simulink model "modos_deslizantes"  (R2025b)
settings: Solver=VariableStepAuto  StartTime=0.0  StopTime=50  RelTol=1e-3
libraries: simulink x1
settings Model: Creator=LENOVO  LastModifiedBy=LENOVO

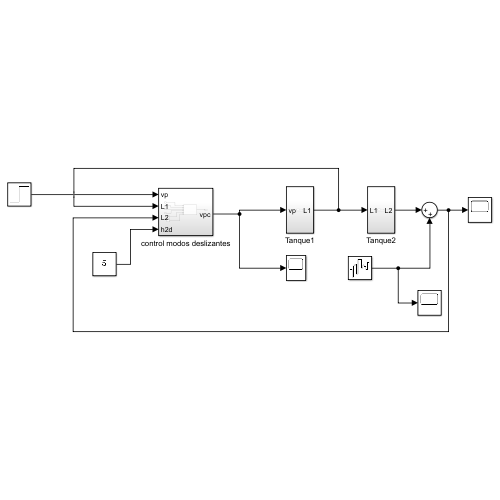
[thumbnail: Simulink's stored preview of the top-level diagram]
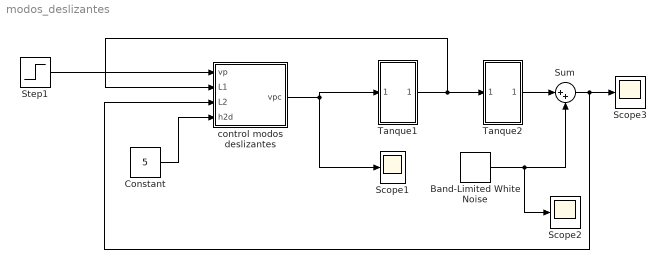
== system modos_deslizantes ==
  Band-Limited White Noise : simulink/Sources/Band-Limited White Noise  Cov=[0.1]  Ts=5  seed=[23341]
  Constant : Constant  Value=5
  Scope1 : Scope
      settings: ActiveDisplayYMinimum=-29.991396434772103  ActiveDisplayYMaximum=28.288118686222941
  Scope2 : Scope
      settings: ActiveDisplayYMinimum=-3.4612563380497452  ActiveDisplayYMaximum=7.7257857094803253  DataLoggingVariableName=ScopeData2
  Scope3 : Scope
      settings: ActiveDisplayYMinimum=-3.4612563380497452  ActiveDisplayYMaximum=7.7257857094803253
  Step1 : Step  After=8  SampleTime=0
  Sum : Sum  Inputs=|++
  Tanque1 : Subsystem
  Tanque2 : Subsystem
  control modos deslizantes : Subsystem
  wires:
  Band-Limited White Noise/1 -> Sum/2, Scope2/1
  control modos deslizantes/1(vpc) -> Tanque1/1(vp), Scope1/1
  Tanque2/1(L2) -> Sum/1
  Sum/1 -> Scope3/1, control modos deslizantes/3(L2)
  Step1/1 -> control modos deslizantes/1(vp)
  Tanque1/1(L1) -> control modos deslizantes/2(L1), Tanque2/1(L1)
  Constant/1 -> control modos deslizantes/4(h2d)

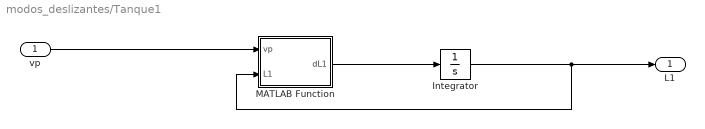
== system modos_deslizantes/Tanque1 ==
  vp : Inport
  Integrator : Integrator
  MATLAB Function : MATLAB Function  TreatAsAtomicUnit=on
  L1 : Outport
  wires:
  Integrator/1 -> L1/1, MATLAB Function/2(L1)
  MATLAB Function/1(dL1) -> Integrator/1
  vp/1 -> MATLAB Function/1(vp)

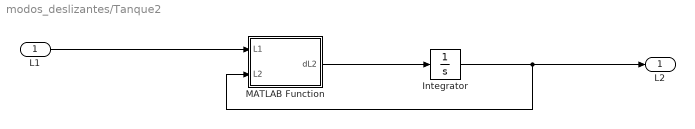
== system modos_deslizantes/Tanque2 ==
  L1 : Inport
  Integrator : Integrator
  MATLAB Function : MATLAB Function  TreatAsAtomicUnit=on
  L2 : Outport
  wires:
  Integrator/1 -> MATLAB Function/2(L2), L2/1
  MATLAB Function/1(dL2) -> Integrator/1
  L1/1 -> MATLAB Function/1(L1)

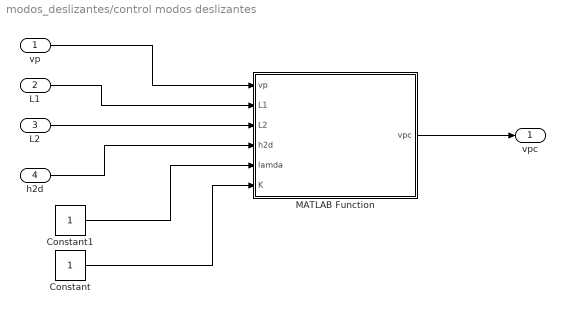
== system modos_deslizantes/control modos deslizantes ==
  vp : Inport
  L1 : Inport  Port=2
  L2 : Inport  Port=3
  h2d : Inport  Port=4
  Constant : Constant
  Constant1 : Constant
  MATLAB Function : MATLAB Function  TreatAsAtomicUnit=on
  vpc : Outport
  wires:
  L1/1 -> MATLAB Function/2(L1)
  MATLAB Function/1(vpc) -> vpc/1
  L2/1 -> MATLAB Function/3(L2)
  vp/1 -> MATLAB Function/1(vp)
  Constant1/1 -> MATLAB Function/5(lamda)
  Constant/1 -> MATLAB Function/6(K)
  h2d/1 -> MATLAB Function/4(h2d)

== matlab function modos_deslizantes/Tanque2/MATLAB Function ==
  data: L1 input; L2 input; dL2 output
function dL2 = fcn(L1, L2)
if L2<0 
   L2=0; 
end
d1=0.635;
a1=pi*d1^2/4;
D2=4.445;
d2=0.47625;
A2=pi*D2^2/4;
a2=pi*d2^2/4;
g=980;

Qin=sqrt(2*g*L1)*a1;
Vout2=sqrt(2*g*L2);
Qout2=Vout2*a2;

dL2 = (Qin-Qout2)/A2;

== matlab function modos_deslizantes/Tanque1/MATLAB Function ==
  data: vp input; dL1 output; L1 input
function dL1 = fcn(vp, L1)

D1=4.445;
d1=0.635;
A1=pi*D1^2/4;
a1=pi*d1^2/4;
Kp=3.3;
g=980;

Qi=vp*Kp;
Vout=sqrt(2*g*L1);
Qout=Vout*a1;

dL1 = (Qi-Qout)/A1;

== matlab function modos_deslizantes/control modos deslizantes/MATLAB Function ==
  data: vp input; L1 input; vpc output; L2 input; h2d input; lamda input; K input
function vpc = fcn(vp,L1,L2,h2d,lamda,K)

x1=L2;
x2=L1;

D1=4.445;
d1=0.635;
A1=pi*D1^2/4;
a1=pi*d1^2/4;
Kp=3.3;
g=980;

D2=4.445;
d2=0.47625;
A2=pi*D2^2/4;
a2=pi*d2^2/4;

B=a1*sqrt(2*g)/A2;
B2=a2*sqrt(2*g)/A2;

y=Kp/A1;
y2=a1*sqrt(2*g)/A1;

if L2<h2d
    vpc=vp;
else

    G=2*sqrt(x2)/(B*y);
    F=B*y2/2 - B*B2*sqrt(x2)/(2*sqrt(x1)) + B2^2/2;
    
    e=x1-h2d;
    de=B*sqrt(x2)-B2*sqrt(x1);
    s=de+lamda*e;
    
    u=G*(-F-lamda*de - K*sign(s));
    if u<-vp
        vpc=0;
    else
        vpc=vp+u;
    end
end
